simulink model "Yolo_test"  (R2024a)
settings: Solver=VariableStepAuto  StartTime=0.0  StopTime=inf  RelTol=1e-3
undefined symbols (not defined in the file or in its folder): Angle, Axis, gray
libraries: robotcorelib x6, eeGeneralControl x2
settings Model: Creator=user  LastModifiedBy=quentinlandon

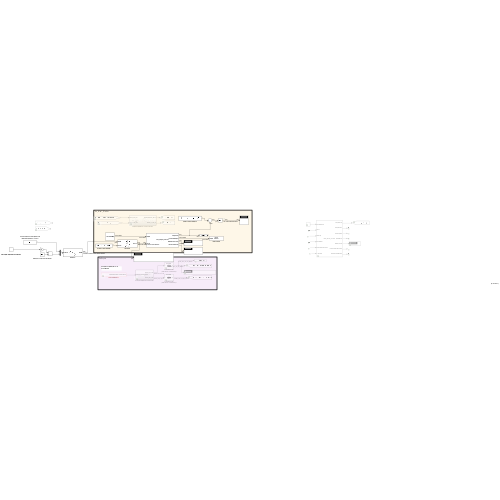
[thumbnail: Simulink's stored preview of the top-level diagram]
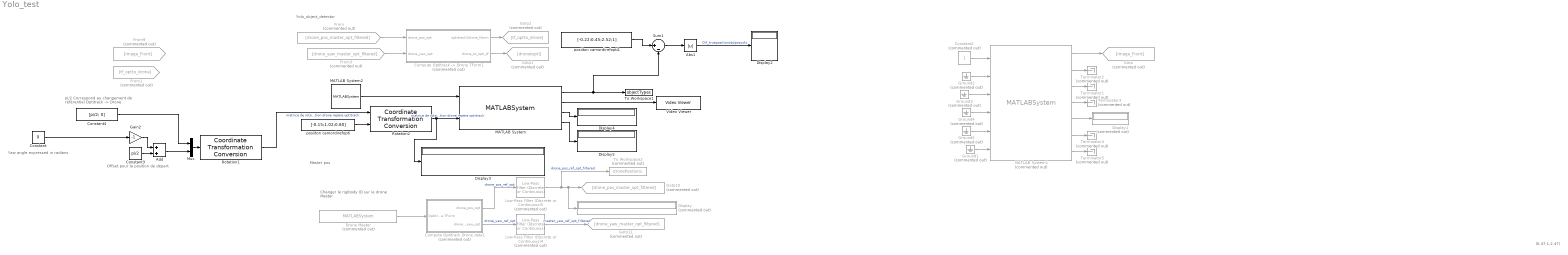
== system Yolo_test ==
  note: Yolo_object_detector
  note: Changer le rigibody ID sur le drone Master
  note: Master pos
  note: (0.47;1;2.47)
  note: pi/2 Correspond au changement de référentiel Optitrack -> Drone
  note: Offset pour la position de départ
  note: Yaw angle expressed in radians
  Abs1 : Abs  SaturateOnIntegerOverflow=off
  Add : Sum
  "Compute Optitrack -> Drone TForm1" : Subsystem  Commented=on
  Compute Optitrack Drone data1 : Subsystem  Commented=on
  Constant : Constant  Value=0
  Constant2 : Constant  Commented=on
  Constant3 : Constant  Value=pi/2
  Constant4 : Constant  Value=[pi/2; 0]
  Display : Display  Commented=on
  Display1 : Display  Commented=on
  Display{2..5} (4 alike) : Display
  Drone Master : MATLABSystem  Commented=on  System=OptilinkSystem  HostIP=10.147.125.15  ClientIP=10.147.125.15  RigidbodyID=1  SimulateUsing=Interpreted execution
      mask Type: OptilinkSystem
      mask Display:
      | disp('OptilinkSystem');
      | port_label('output',1,'Drones data');
  From : From  Commented=on  GotoTag=drone_pos_master_opt_filtered
  From1 : From  Commented=on  GotoTag=tf_optto_drone
  From3 : From  Commented=on  GotoTag=drone_yaw_master_opt_filtered
  From9 : From  Commented=on  GotoTag=Image_Front
  Gain2 : Gain  Gain=-1
  Goto : Goto  Commented=on  GotoTag=Image_Front
  Goto1 : Goto  Commented=on  GotoTag=dronetopti
  Goto10 : Goto  Commented=on  GotoTag=drone_pos_master_opt_filtered
  Goto11 : Goto  Commented=on  GotoTag=drone_yaw_master_opt_filtered
  Goto2 : Goto  Commented=on  GotoTag=tf_optto_drone
  Ground{1..5} (5 alike) : Ground  Commented=on
  Low-Pass Filter (Discrete or Continuous)4 : eeGeneralControl/Low-Pass Filter (Discrete or Continuous)  Commented=on  K=1  T=1.5  B=inf  A=-inf  init_option=Inherited from block input  x0=0  Ts=-1
  Low-Pass Filter (Discrete or Continuous)5 : eeGeneralControl/Low-Pass Filter (Discrete or Continuous)  Commented=on  K=1  T=1.5  B=inf  A=-inf  init_option=Inherited from block input  x0=0  Ts=-1
  MATLAB System : MATLABSystem  System=Yolo_Object_Detector  SimulateUsing=Interpreted execution
      mask Type: Yolo_Object_Detector
      mask Display:
      | disp('Yolo_Object_Detector');
      | port_label('input',1,'Image');
      | port_label('input',2,'Tform');
      | port_label('output',1,'ObjectPos');
      | port_label('output',2,'AnnotatedImage');
      | port_label('output',3,'BBoxDimensions');
      | port_label('output',4,'CamCoordinates');
  MATLAB System1 : MATLABSystem  Commented=on  System=Tello_drone_control  droneIP=127.0.0.1  SimulateUsing=Interpreted execution
      mask Type: Tello_drone_control
      mask Display:
      | disp('Tello_drone_control');
      | port_label('input',1,'enableVideo');
      | port_label('input',2,'tkoff');
      | port_label('input',3,'landing');
      | port_label('input',4,'enableRC');
      | port_label('input',5,'cmdVideoDirection');
      | port_label('input',6,'rcspeeds');
      | port_label('output',1,'imageFront');
      | port_label('output',2,'imageDown');
      | port_label('output',3,'Eulerangles');
      | port_label('output',4,'speedXYZ');
      | port_label('output',5,'batteryLevel');
      | port_label('output',6,'currentVideoDirection');
      | port_label('output',7,'hasTakenOffStatus');
  MATLAB System2 : MATLABSystem  System=cameramac  SimulateUsing=Interpreted execution
      mask Type: cameramac
      mask Display:
      | disp('cameramac');
      | port_label('output',1,'img');
  Mux : Mux  Inputs=2
  Rotation1 : robotcorelib/Coordinate Transformation Conversion  InputRepresentation=Euler Angles  InputEulerSequence=XYZ  ShowTrVecInputPort=off  OutputRepresentation=Rotation Matrix  OutputEulerSequence=ZYX  ShowTrVecOutputPort=off  SimulateUsing=Code generation
      settings: LibrarySourceBlock=uavutilslib/Coordinate Transformation Conversion
  Rotation2 : robotcorelib/Coordinate Transformation Conversion  InputRepresentation=Rotation Matrix  InputEulerSequence=XYZ  ShowTrVecInputPort=on  OutputRepresentation=Homogeneous Transformation  OutputEulerSequence=ZYX  ShowTrVecOutputPort=off  SimulateUsing=Code generation
      settings: LibrarySourceBlock=uavutilslib/Coordinate Transformation Conversion
  Sum1 : Sum  Inputs=|+-
  Terminator{1..5} (5 alike) : Terminator  Commented=on
  To Workspace1 : ToWorkspace  VariableName=objectTypes  SaveFormat=Structure With Time  SampleTime=-1
  To Workspace2 : ToWorkspace  Commented=on  VariableName=dronePositions  SaveFormat=Structure With Time  SampleTime=-1
  Video Viewer : VideoViewer  colormapValue=gray(256)  FigPos=[166 838 752 592]
  posiiton camordirefopti : Constant  Value=[-0.15;1.02;0.80]
  posiiton camordirefopti1 : Constant  Value=[-0.22;0.45;2.52;1]
  wires:
  MATLAB System/2 -> Video Viewer/1
  MATLAB System2/1 -> MATLAB System/1
  Low-Pass Filter (Discrete or Continuous)4/1 -> Goto11/1  "master_yaw_ref_opt_filtered"
  Low-Pass Filter (Discrete or Continuous)5/1 -> To Workspace2/1, Display/1, Goto10/1  "drone_pos_ref_opt_filtered"
  Compute Optitrack Drone data1/2(drone_yaw_opt) -> Low-Pass Filter (Discrete or Continuous)4/1  "drone_yaw_ref_opt"
  Drone Master/1 -> Compute Optitrack Drone data1/1(Optitrack Drone TForm)
  Compute Optitrack Drone data1/1(drone_pos_opt) -> Low-Pass Filter (Discrete or Continuous)5/1  "drone_pos_ref_opt"
  Constant2/1 -> MATLAB System1/1
  MATLAB System1/2 -> Terminator2/1
  MATLAB System1/3 -> Terminator1/1
  MATLAB System1/4 -> Terminator3/1
  Ground1/1 -> MATLAB System1/6
  Ground3/1 -> MATLAB System1/3
  MATLAB System1/5 -> Display1/1
  MATLAB System1/7 -> Terminator5/1
  Ground4/1 -> MATLAB System1/4
  Ground2/1 -> MATLAB System1/2
  MATLAB System1/6 -> Terminator4/1
  Ground5/1 -> MATLAB System1/5
  MATLAB System1/1 -> Goto/1
  From/1 -> "Compute Optitrack -> Drone TForm1"/1(drone_pos_opt)
  From3/1 -> "Compute Optitrack -> Drone TForm1"/2(drone_yaw_opt)
  "Compute Optitrack -> Drone TForm1"/1(optitrack2drone_tform) -> Goto2/1
  posiiton camordirefopti1/1 -> Sum1/1
  "Compute Optitrack -> Drone TForm1"/2(drone_to_opti_tf) -> Goto1/1
  Sum1/1 -> Abs1/1
  Abs1/1 -> Display2/1  "Dif_truepositionobj/posyolo"
  MATLAB System/1 -> To Workspace1/1, Sum1/2
  Constant/1 -> Gain2/1
  Add/1 -> Mux/2
  Mux/1 -> Rotation1/1
  Gain2/1 -> Add/1
  Constant4/1 -> Mux/1
  Constant3/1 -> Add/2
  Rotation1/1 -> Rotation2/1  "matrice de rotation drone repère optitrack"
  posiiton camordirefopti/1 -> Rotation2/2
  Rotation2/1 -> Display3/1, MATLAB System/2  "matrice de rotation drone repère optitrack"
  MATLAB System/3 -> Display4/1
  MATLAB System/4 -> Display5/1

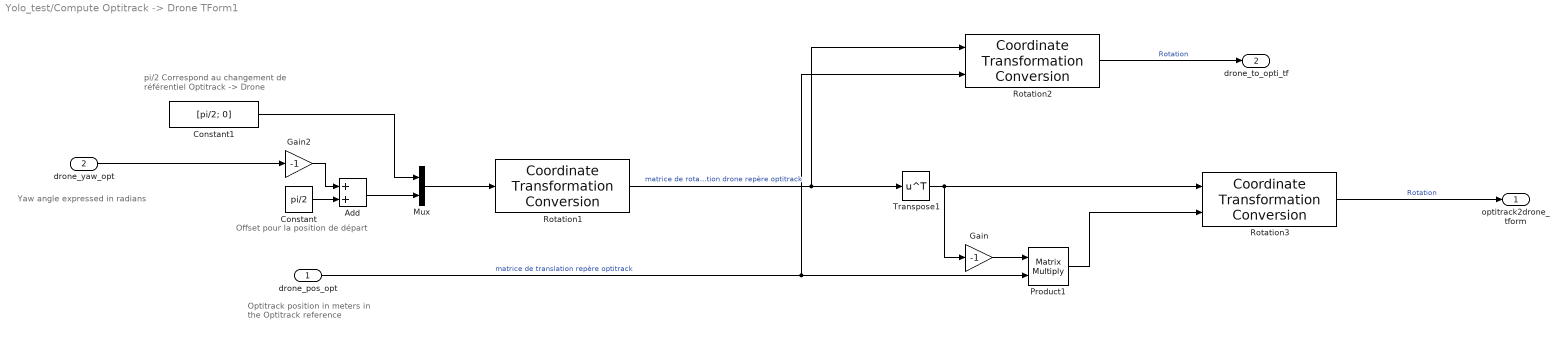
== system Yolo_test/Compute Optitrack -> Drone TForm1 ==
  note: Yaw angle expressed in radians
  note: Offset pour la position de départ
  note: pi/2 Correspond au changement de référentiel Optitrack -> Drone
  note: Optitrack position in meters
      | in the Optitrack reference
  drone_pos_opt : Inport
  drone_yaw_opt : Inport  Port=2
  Add : Sum
  Constant : Constant  Value=pi/2
  Constant1 : Constant  Value=[pi/2; 0]
  Gain : Gain  Gain=-1
  Gain2 : Gain  Gain=-1
  Mux : Mux  Inputs=2
  Product1 : Product  Multiplication=Matrix(*)
  Rotation1 : robotcorelib/Coordinate Transformation Conversion  InputRepresentation=Euler Angles  InputEulerSequence=XYZ  ShowTrVecInputPort=off  OutputRepresentation=Rotation Matrix  OutputEulerSequence=ZYX  ShowTrVecOutputPort=off  SimulateUsing=Code generation
      settings: LibrarySourceBlock=uavutilslib/Coordinate Transformation Conversion
  Rotation2 : robotcorelib/Coordinate Transformation Conversion  InputRepresentation=Rotation Matrix  InputEulerSequence=XYZ  ShowTrVecInputPort=on  OutputRepresentation=Homogeneous Transformation  OutputEulerSequence=ZYX  ShowTrVecOutputPort=off  SimulateUsing=Code generation
      settings: LibrarySourceBlock=uavutilslib/Coordinate Transformation Conversion
  Rotation3 : robotcorelib/Coordinate Transformation Conversion  InputRepresentation=Rotation Matrix  InputEulerSequence=XYZ  ShowTrVecInputPort=on  OutputRepresentation=Homogeneous Transformation  OutputEulerSequence=ZYX  ShowTrVecOutputPort=off  SimulateUsing=Code generation
      settings: LibrarySourceBlock=uavutilslib/Coordinate Transformation Conversion
  Transpose1 : Math  Operator=transpose
  optitrack2drone_tform : Outport
  drone_to_opti_tf : Outport  Port=2
  wires:
  Add/1 -> Mux/2
  Transpose1/1 -> Rotation3/1, Gain/1
  Constant/1 -> Add/2
  Gain2/1 -> Add/1
  Product1/1 -> Rotation3/2
  Constant1/1 -> Mux/1
  Rotation1/1 -> Rotation2/1, Transpose1/1  "matrice de rotation drone repère optitrack"
  Gain/1 -> Product1/1
  Mux/1 -> Rotation1/1
  drone_pos_opt/1 -> Rotation2/2, Product1/2  "matrice de translation repère optitrack"
  drone_yaw_opt/1 -> Gain2/1
  Rotation3/1 -> optitrack2drone_tform/1  "Rotation"
  Rotation2/1 -> drone_to_opti_tf/1  "Rotation"

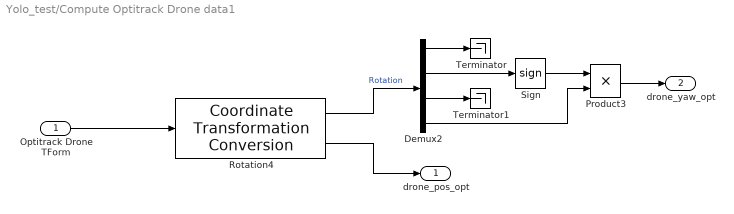
== system Yolo_test/Compute Optitrack Drone data1 ==
  Optitrack Drone TForm : Inport
  Demux2 : Demux
  Product3 : Product
  Rotation4 : robotcorelib/Coordinate Transformation Conversion  InputRepresentation=Homogeneous Transformation  InputEulerSequence=XYZ  ShowTrVecInputPort=on  OutputRepresentation=Axis-Angle  OutputEulerSequence=XYZ  ShowTrVecOutputPort=on  SimulateUsing=Code generation
      settings: LibrarySourceBlock=uavutilslib/Coordinate Transformation Conversion
  Sign : Signum
  Terminator : Terminator
  Terminator1 : Terminator
  drone_pos_opt : Outport
  drone_yaw_opt : Outport  Port=2
  wires:
  Rotation4/2 -> drone_pos_opt/1
  Demux2/4 -> Product3/2
  Rotation4/1 -> Demux2/1  "Rotation"
  Sign/1 -> Product3/1
  Demux2/2 -> Sign/1
  Product3/1 -> drone_yaw_opt/1
  Optitrack Drone TForm/1 -> Rotation4/1
  Demux2/3 -> Terminator1/1
  Demux2/1 -> Terminator/1
